simulink model "penduloinvertido"  (R2019b)
settings: Solver=VariableStepAuto  StartTime=0.0  StopTime=5  RelTol=1e-3
values from neighbouring files (symbols this model uses):
  cr = 0.05    [confusion.m]    (also in main.m; tarea3.m)
  eq = solve(H)    [main.m]    (also in tarea3.m)
  g = 9.81    [confusion.m]    (also in main.m; tarea3.m)
  J = m*(l^2)    (= 0.39375)    [confusion.m]    (also in main.m; tarea3.m)
  K_pd = 14    [main.m]    (also in tarea3.m = 40)
  l = 0.75    [confusion.m]    (also in main.m; tarea3.m)
  m = 0.7    [confusion.m]    (also in main.m; tarea3.m)
  p = double(solve(H==0))    [confusion.m]    (also in main.m = 10; tarea3.m = 10)
settings Model: Creator=Gamer  LastModifiedBy=Gamer
settings DataIOCC: Refine=10

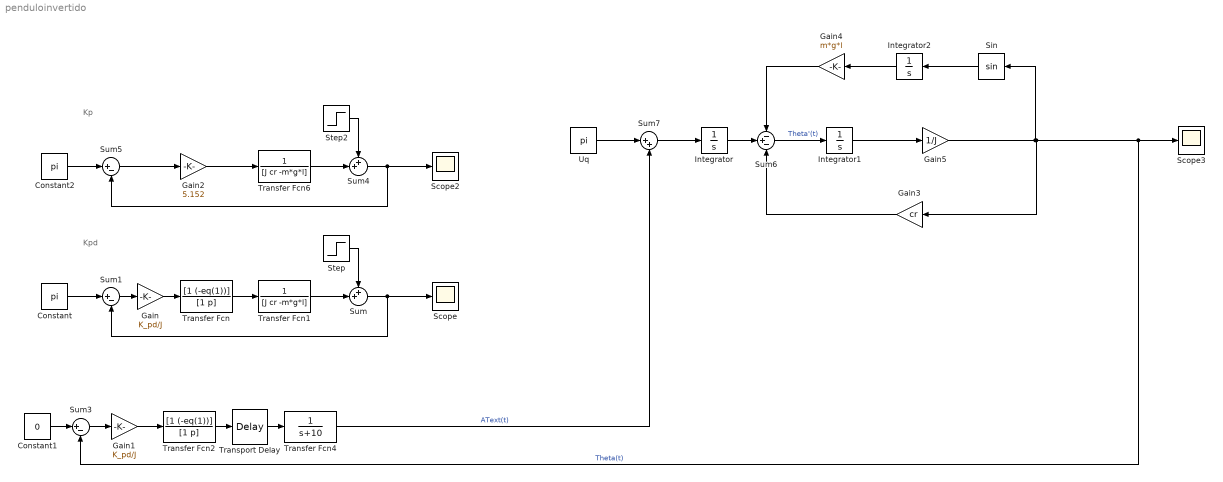
== system penduloinvertido ==
  note: Kpd
  note: Kp
  Constant : Constant  Value=pi
  Constant1 : Constant  Value=0
  Constant2 : Constant  Value=pi
  Gain : Gain  Gain=K_pd/J
  Gain1 : Gain  Gain=K_pd/J
  Gain2 : Gain  Gain=5.152
  Gain3 : Gain  Gain=cr
  Gain4 : Gain  Gain=m*g*l
  Gain5 : Gain  Gain=1/J
  Integrator : Integrator
  Integrator1 : Integrator
  Integrator2 : Integrator
  Scope : Scope
  Scope2 : Scope
  Scope3 : Scope
  Sin : Trigonometry
  Step : Step  SampleTime=0
  Step2 : Step  SampleTime=0
  Sum : Sum  Inputs=++|
  Sum1 : Sum  Inputs=|+-
  Sum3 : Sum  Inputs=|+-
  Sum4 : Sum  Inputs=++|
  Sum5 : Sum  Inputs=|+-
  Sum6 : Sum  Inputs=-+-
  Sum7 : Sum  Inputs=|++
  Transfer Fcn : TransferFcn  Numerator=[1 (-eq(1))]  Denominator=[1 p]
  Transfer Fcn1 : TransferFcn  Denominator=[J cr -m*g*l]
  Transfer Fcn2 : TransferFcn  Numerator=[1 (-eq(1))]  Denominator=[1 p]
  Transfer Fcn4 : TransferFcn  Denominator=[1 10]
  Transfer Fcn6 : TransferFcn  Denominator=[J cr -m*g*l]
  Transport Delay : TransportDelay  DelayTime=0.1
  Uq : Constant  Value=pi
  wires:
  Transfer Fcn/1 -> Transfer Fcn1/1
  Transfer Fcn1/1 -> Sum/2
  Sum/1 -> Scope/1, Sum1/2
  Constant/1 -> Sum1/1
  Sum1/1 -> Gain/1
  Gain/1 -> Transfer Fcn/1
  Step/1 -> Sum/1
  Constant1/1 -> Sum3/1
  Step2/1 -> Sum4/1
  Transfer Fcn6/1 -> Sum4/2
  Sum5/1 -> Gain2/1
  Constant2/1 -> Sum5/1
  Sum4/1 -> Scope2/1, Sum5/2
  Gain2/1 -> Transfer Fcn6/1
  Transport Delay/1 -> Transfer Fcn4/1
  Transfer Fcn2/1 -> Transport Delay/1
  Sum3/1 -> Gain1/1
  Gain1/1 -> Transfer Fcn2/1
  Gain5/1 -> Sin/1, Sum3/2, Scope3/1, Gain3/1  "Theta(t)"
  Gain3/1 -> Sum6/3
  Gain4/1 -> Sum6/1
  Sin/1 -> Integrator2/1
  Uq/1 -> Sum7/1
  Integrator2/1 -> Gain4/1
  Integrator1/1 -> Gain5/1
  Integrator/1 -> Sum6/2
  Sum6/1 -> Integrator1/1  "Theta'(t)"
  Transfer Fcn4/1 -> Sum7/2  "AText(t)"
  Sum7/1 -> Integrator/1
